simulink library "hcu_lib"  (R2021b)
settings: Solver=VariableStepAuto  StartTime=0.0  StopTime=10.0  RelTol=1e-3
undefined symbols (not defined in the file): ENUM_FAULTSTATE_FAIL, ENUM_FAULTSTATE_INDETERMINATE, ENUM_FAULTSTATE_PASS, EPSILON, FALSE, KPH2MPH, KPH2MPS, KXX2XX, MPH2KPH, MPS2KPH, ONE_INT16, ONE_INT32, RADPS2RPM, RPM2RADPS, slcm, TRUE, UNDEFINED_VALUE, XX2KXX, ZERO_FLOAT, ZERO_INT, ZERO_INT16, ZERO_INT32
libraries: $bdroot x31, simulink x10, afl x1
(part 3 of 3)

== stateflow chart hcu_lib/Basic_Blocks/Minutes_Counter/Scheduler ==
  state trigger_1min
    (default) -> (junction 63) : {
        | counter = 0;
        | }
    trigger_1min -> (junction 63)
    (junction 63) -> (junction 41) [order 1] : [trigger]
    (junction 63) -> (junction 68) [order 2] : {
        | trig_1min = 0;
        | }
    (junction 41) -> (junction 1) : {
        | counter++;
        | }
    (junction 1) -> (junction 8) [order 1] : [counter%%uint32((60*1/task_time_s)) == 0]  /* 1min trigger */
    (junction 1) -> (junction 5) [order 2] : {
        | trig_1min = 0;
        | }
    (junction 8) -> (junction 9) : {
        | trig_1min = 1;
        | counter = 0;
        | }
  data: counter local uint32 size=1; task_time_s input; trigger input; trig_1min output boolean

== stateflow chart hcu_lib/Basic_Blocks/Seconds_Counter/Scheduler ==
  state trigger_1sec
    (default) -> (junction 63) : {
        | counter = 0;
        | }
    trigger_1sec -> (junction 63)
    (junction 63) -> (junction 41) [order 1] : [trigger]
    (junction 63) -> (junction 68) [order 2] : {
        | trig_1sec = 0;
        | }
    (junction 41) -> (junction 1) : {
        | counter++;
        | }
    (junction 1) -> (junction 8) [order 1] : [counter%%uint32(1/task_time_s) == 0]  /* 1sec trigger */
    (junction 1) -> (junction 5) [order 2] : {
        | trig_1sec = 0;
        | }
    (junction 8) -> (junction 9) : {
        | trig_1sec = 1;
        | counter = 0;
        | }
  data: counter local uint32 size=1; task_time_s input; trigger input; trig_1sec output boolean

== stateflow chart hcu_lib/Basic_Blocks/RangeTimer/Scheduler ==
  state trigger_1sec
    (default) -> (junction 63) : {
        | counter = 0;
        | }
    trigger_1sec -> (junction 63)
    (junction 63) -> (junction 41) [order 1] : [trigger]
    (junction 63) -> (junction 68) [order 2] : {
        | trig_1sec = 0;
        | }
    (junction 41) -> (junction 1) : {
        | counter++;
        | }
    (junction 1) -> (junction 8) [order 1] : [counter%%uint32(1/task_time_s) == 0]  /* 1sec trigger */
    (junction 1) -> (junction 5) [order 2] : {
        | trig_1sec = 0;
        | }
    (junction 8) -> (junction 9) : {
        | trig_1sec = 1;
        | counter = 0;
        | }
  data: counter local uint32 size=1; task_time_s input; trigger input; trig_1sec output boolean

== stateflow chart hcu_lib/Signal_Process_Blocks/latching_fault_filter/lff_ctl ==
  (default) -> (junction 9)
  (junction 9) -> (junction 13) [order 1] : [i_fault]
      | {count+=inc;}
  (junction 9) -> (junction 13) [order 2] : {count-=dec;}
  (junction 13) -> (junction 10)
  (junction 10) -> (junction 11) [order 1] : [count>=sat]
      | {count=sat;
      | fault_flg=1;}
  (junction 10) -> (junction 11) [order 2] : [count<=0]
      | {count=0;}
  (junction 10) -> (junction 11) [order 3]
  (junction 11) -> (junction 12) : {ff_count = count;}
  data: sat input uint8; inc input uint8; dec input uint8; i_fault input boolean; fault_flg output boolean =0; ff_count output uint8; count local int16 =0

== stateflow chart hcu_lib/Signal_Process_Blocks/latching fault filter reinit/lff_ctl ==
  (default) -> (junction 25)
  (junction 25) -> (junction 27) [order 1] : [reinit]
  (junction 25) -> (junction 20) [order 2]
  (junction 27) -> (junction 28) : {fault_flg = FALSE;
      |  count = 0;}
  (junction 20) -> (junction 29) [order 1] : [i_fault]
  (junction 20) -> (junction 24) [order 2] : {count-=dec;}
  (junction 29) -> (junction 30) : {count+=inc;}
  (junction 30) -> (junction 24)
  (junction 24) -> (junction 21)
  (junction 21) -> (junction 31) [order 1] : [count >= sat]
  (junction 21) -> (junction 26) [order 2]
  (junction 31) -> (junction 32) : {count = sat;
      | fault_flg = TRUE;}
  (junction 26) -> (junction 34) [order 1] : [count <= 0]
  (junction 26) -> (junction 22) [order 2]
  (junction 34) -> (junction 33) : {count = 0;}
  (junction 33) -> (junction 22)
  (junction 32) -> (junction 33)
  (junction 28) -> (junction 32)
  (junction 22) -> (junction 23) : {ff_count = count;}
  data: sat input uint8; inc input uint8; dec input uint8; i_fault input boolean; fault_flg output boolean =0; ff_count output uint8; count local int16 =0; TRUE parameter boolean; FALSE parameter boolean; reinit input boolean
